simulink model "f_tau_model"  (R2023b)
settings: Solver=VariableStepAuto  StartTime=0.0  StopTime=10.0  RelTol=1e-3
values from neighbouring files (symbols this model uses):
  alpha_k = constantes(14)    [calculaMatrizesModelo.m]    (also in integracaoNumerica.m = c(12); simulaModeloSimulink.m; simulaTrajetoriaSimulink.m)
  alpha_s = constantes(13)    [calculaMatrizesModelo.m]    (also in integracaoNumerica.m = c(11); simulaModeloSimulink.m; simulaTrajetoriaSimulink.m)
  f_k = constantes(12)    [calculaMatrizesModelo.m]    (also in simulaModeloSimulink.m; simulaTrajetoriaSimulink.m)
  f_s = constantes(11)    [calculaMatrizesModelo.m]    (also in simulaModeloSimulink.m; simulaTrajetoriaSimulink.m)
  g = 9.81    [calculaMatrizesModelo.m]    (also in integracaoNumerica.m; simulaModeloSimulink.m; simulaTrajetoriaSimulink.m)
  m = m_c + 2*m_w    [calculaMatrizesModelo.m]    (also in integracaoNumerica.m = mc + 2*mw; simulaModeloSimulink.m; simulaTrajetoriaSimulink.m)
settings Model: Creator=Gabriel Sousa  LastModifiedBy=Gabriel Sousa

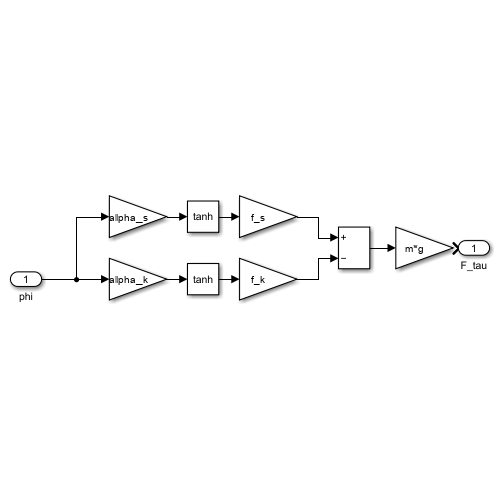
[thumbnail: Simulink's stored preview of the top-level diagram]
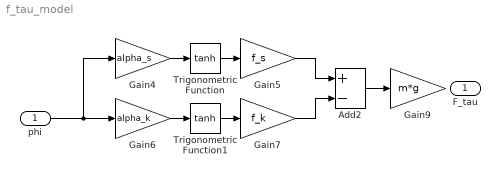
== system f_tau_model ==
  phi : Inport
  Add2 : Sum  Inputs=+-
  Gain4 : Gain  Gain=alpha_s
  Gain5 : Gain  Gain=f_s
  Gain6 : Gain  Gain=alpha_k
  Gain7 : Gain  Gain=f_k
  Gain9 : Gain  Gain=m*g
  Trigonometric Function : Trigonometry  Operator=tanh
  Trigonometric Function1 : Trigonometry  Operator=tanh
  F_tau : Outport
  wires:
  Gain4/1 -> Trigonometric Function/1
  Trigonometric Function1/1 -> Gain7/1
  Gain7/1 -> Add2/2
  Add2/1 -> Gain9/1
  phi/1 -> Gain4/1, Gain6/1
  Gain6/1 -> Trigonometric Function1/1
  Gain5/1 -> Add2/1
  Trigonometric Function/1 -> Gain5/1
